simulink model "Droop_test2"  (R2024a)
settings: Solver=VariableStepAuto  StartTime=0.0  StopTime=1  RelTol=1e-3
InitFcn:
  |  if any(exist('rtifpga_mdlclblib', 'file') ~= 0), rtifpga_mdlclblib('Init', bdroot); end,
  | Ts  = 10e-6;
  | 
  | Vpeak = 170;
  | Vnom = Vpeak*sqrt(3)/sqrt(2);
  | Fnom = 60;
  | w_rad  = 2*pi*Fnom;
  | 
  | Vdc2 = 300;
  | 
  | % LC filter for DG1
  | L11 = 5e-03;
  | Cf1 = 30e-06;
  | Rc1 = 0.5;           % Damping series-resistor
  | RL1 = 0.9;        % Inductor ESR
  | L22=1e-12;
  | % LC filter for DG2
  | L12 = 5e-03;
  | Cf2 = 10e-06;
  | Rc2 = 0.5;           % Damping series-resistor
  | RL2 = 0.9;        % Inductor ESR
  | 
  | Pnom = 1000;
libraries: spsThreePhaseSeriesRLCBranchLib x5, spsabctoAlphaBetaZeroLib x4, spsGroundLib x3, spsFirstOrderFilterLib x2, spsThreePhaseVIMeasurementLib x2, spsabctodq0Lib x2, spsDCVoltageSourceLib x1, spsPLL3phLib x1, spsThreePhaseBreakerLib x1, spsUniversalBridgeLib x1, sps_lib x1
settings Model: Creator=azare  LastModifiedBy=nicho
settings OptimizationCC: ReuseModelBlockBuffer=off
settings RTWCC: GenCodeOnly=on  GPUComputeCapability=3.5
settings GRTTargetCC: OptimizeReductions=on

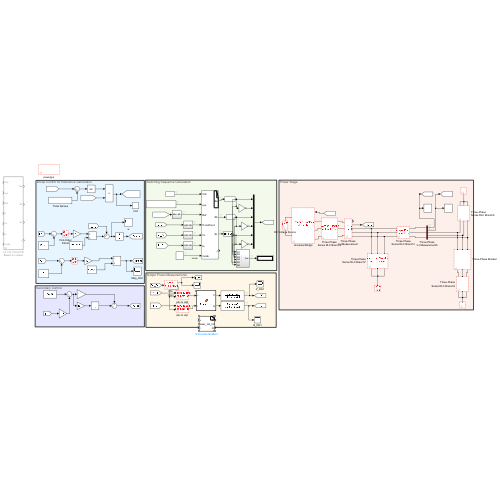
[thumbnail: Simulink's stored preview of the top-level diagram]
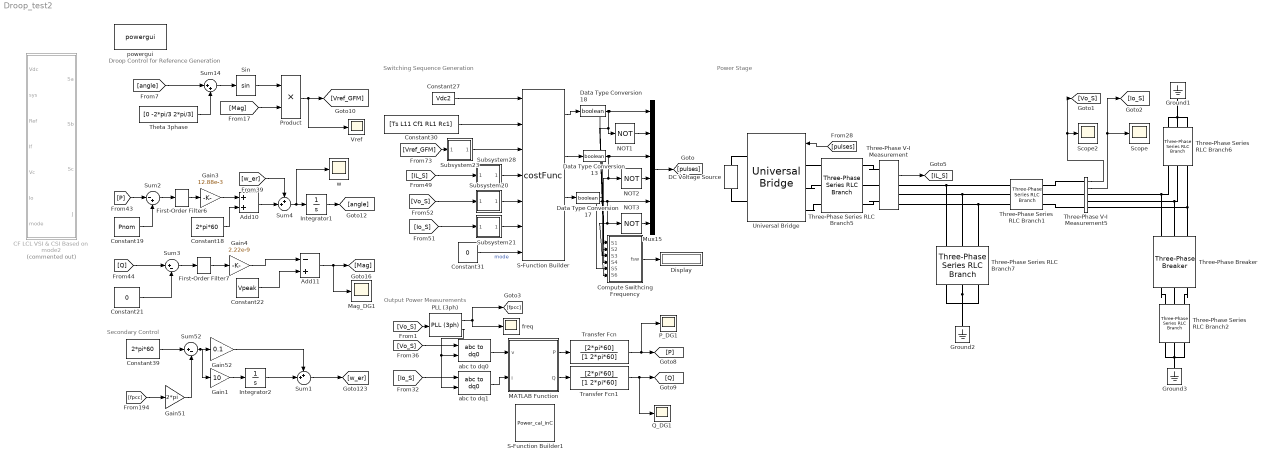
== system Droop_test2 ==
  note: Power Stage
  note: Output Power Measurements
  note: Switching Sequence Generation
  note: Droop Control for Reference Generation
  note: Secondary Control
  Add10 : Sum
  Add11 : Sum  Inputs=-+
  CF LCL VSI & CSI Based on mode2 : MATLAB Function  Commented=on  TreatAsAtomicUnit=on
  Compute Swithcing Frequency : Subsystem
  Constant18 : Constant  Value=2*pi*60
  Constant19 : Constant  Value=Pnom
  Constant21 : Constant  Value=0
  Constant22 : Constant  Value=Vpeak
  Constant27 : Constant  Value=Vdc2
  Constant30 : Constant  Value=[Ts L11 Cf1 RL1 Rc1]
  Constant31 : Constant  Value=0
  Constant39 : Constant  Value=2*pi*60
  DC Voltage Source : spsDCVoltageSourceLib/DC Voltage Source  Amplitude=Vdc2  Measurements=None
  Data Type Conversion13 : DataTypeConversion  OutDataTypeStr=boolean
  Data Type Conversion17 : DataTypeConversion  OutDataTypeStr=boolean
  Data Type Conversion18 : DataTypeConversion  OutDataTypeStr=boolean
  Display : Display
  First-Order Filter6 : spsFirstOrderFilterLib/First-Order Filter  FilterType=Lowpass  Tc=12.5e-3  Ts=0  Initialize=on  Vac_Init=[0, 0, 60]  Vdc_Init=0  PlotResponse=off  FreqRange="[0,  200,  1]"
  First-Order Filter7 : spsFirstOrderFilterLib/First-Order Filter  FilterType=Lowpass  Tc=12.5e-3  Ts=0  Initialize=on  Vac_Init=[0, 0, 60]  Vdc_Init=0  PlotResponse=off  FreqRange="[0,  200,  1]"
  Gain1 : Gain  Gain=10
  Gain3 : Gain  Gain=12.88e-3
  Gain4 : Gain  Gain=2.22e-9
  Gain51 : Gain  Gain=2*pi
  Gain52 : Gain  Gain=0.1
  Ground1 : spsGroundLib/Ground  LConnTagsString=a
  Ground2 : spsGroundLib/Ground  LConnTagsString=a
  Ground3 : spsGroundLib/Ground  LConnTagsString=a
  Integrator1 : Integrator
  Integrator2 : Integrator
  MATLAB Function : MATLAB Function  TreatAsAtomicUnit=on
  Mag_DG1 : Scope
  Mux15 : Mux  Inputs=6
  NOT1 : Logic  Operator=NOT  IconShape=distinctive  AllPortsSameDT=off  OutDataTypeStr=boolean
  NOT2 : Logic  Operator=NOT  IconShape=distinctive  AllPortsSameDT=off  OutDataTypeStr=boolean
  NOT3 : Logic  Operator=NOT  IconShape=distinctive  AllPortsSameDT=off  OutDataTypeStr=boolean
  PLL (3ph) : spsPLL3phLib/PLL (3ph)  Fmin=45  Par_Init=[0, 60]  ParK=[180, 3200, 1]  TcD=1e-4  MaxRateChangeFreq=12  FilterCutOffFreq=25  Ts=0  AGC=on
  P_DG1 : Scope
  Product : Product
  Q_DG1 : Scope
  S-Function Builder : S-Function  FunctionName=costFunc  SFunctionModules=costFunc_wrapper.c  SFunctionDeploymentMode=off  EnableBusSupport=off  mask(S-Function Builder){}
      mask help: Simulink:masks:SFunctionBuilder_MD
      mask init:
      | val = [[.9  0.75 0.75 1 1 .9 .9 1]',[1 1 0.75 0.75 .9 .9 1 .9]'];try , sys = get_param(gcb,'SfunBuilderFcnName');if isempty(sys), sys = get_param(gcb,'FunctionName'); end,catch, sys = get_param(gcb,'FunctionName'); end
      settings: CopyFcn=set_param(gcbh,'LinkStatus','none')  OpenFcn=sfunctionwizard(gcbh)
      mask Display:
      | plot(val(:,1),val(:,2))
      | disp(sys)
      | port_label('input',1,sprintf('%s', 'Vdc'),'interpreter','tex')
      | port_label('input',2,sprintf('%s', 'sys'),'interpreter','tex')
      | port_label('input',3,sprintf('%s', 'Ref'),'interpreter','tex')
      | port_label('input',4,sprintf('%s', 'If'),'interpreter','tex')
      | port_label('input',5,sprintf('%s', 'Vc'),'interpreter','tex')
      | port_label('input',6,sprintf('%s', 'Io'),'interpreter','tex')
      | port_label('input',7,sprintf('%s', 'mode'),'interpreter','tex')
      | port_label('output',1,sprintf('%s', 'Sa'),'interpreter','tex')
      | port_label('output',2,sprintf('%s', 'Sb'),'interpreter','tex')
      | port_label('output',3,sprintf('%s', 'Sc'),'interpreter','tex')
      | port_label('output',4,sprintf('%s', 'J'),'interpreter','tex')
  S-Function Builder1 : S-Function  FunctionName=Power_cal_inC  SFunctionModules=Power_cal_inC_wrapper.c  SFunctionDeploymentMode=off  EnableBusSupport=off  mask(S-Function Builder){}
      mask help: Simulink:masks:SFunctionBuilder_MD
      mask init: same as Droop_test2/S-Function Builder
      settings: CopyFcn=set_param(gcbh,'LinkStatus','none')  OpenFcn=sfunctionwizard(gcbh)
      mask Display: plot(val(:,1),val(:,2)),disp(sys),port_label('input',1,'v'),port_label('input',2,'i'),port_label('output',1,'P'),port_label('output',2,'Q')
  Scope : Scope
  Scope2 : Scope
  Sin : Trigonometry
  Subsystem20 : Subsystem
  Subsystem21 : Subsystem
  Subsystem23 : Subsystem
  Subsystem28 : Subsystem
  Sum1 : Sum  Inputs=++|
  Sum14 : Sum  Inputs=|++
  Sum2 : Sum  Inputs=|-+
  Sum3 : Sum  Inputs=|+-
  Sum4 : Sum  Inputs=++|
  Sum52 : Sum  Inputs=|+-
  Theta 3phase : Constant  Value=[0 -2*pi/3 2*pi/3]
  Three-Phase Series RLC Branch1 : spsThreePhaseSeriesRLCBranchLib/Three-Phase Series RLC Branch  LConnTagsString=A|B|C  RConnTagsString=A|B|C  BranchType=RL  Resistance=0.05  Inductance=0.5e-3  Capacitance=0  Measurements=None
  Three-Phase Series RLC Branch2 : spsThreePhaseSeriesRLCBranchLib/Three-Phase Series RLC Branch  LConnTagsString=A|B|C  RConnTagsString=A|B|C  BranchType=R  Resistance=43.35  Inductance=1e-3  Capacitance=10e-6  Measurements=None
  Three-Phase Series RLC Branch5 : spsThreePhaseSeriesRLCBranchLib/Three-Phase Series RLC Branch  LConnTagsString=A|B|C  RConnTagsString=A|B|C  BranchType=RL  Resistance=RL1  Inductance=L11  Capacitance=0  Measurements=None
  Three-Phase Series RLC Branch6 : spsThreePhaseSeriesRLCBranchLib/Three-Phase Series RLC Branch  LConnTagsString=A|B|C  RConnTagsString=A|B|C  BranchType=R  Resistance=43.35  Inductance=1e-3  Capacitance=10e-6  Measurements=None
  Three-Phase Series RLC Branch7 : spsThreePhaseSeriesRLCBranchLib/Three-Phase Series RLC Branch  LConnTagsString=A|B|C  RConnTagsString=A|B|C  BranchType=RC  Resistance=Rc1  Inductance=1e-3  Capacitance=Cf1  Measurements=None
  Three-Phase V-I Measurement : spsThreePhaseVIMeasurementLib/Three-Phase V-I Measurement  VoltageMeasurement=phase-to-ground  SetLabelV=off  LabelV=Vabc  Vpu=off  VpuLL=off  CurrentMeasurement=yes  SetLabelI=off  LabelI=Iabc  Ipu=off  Pbase=100e6  Vbase=500e3  OutputType=Complex  PhasorSimulation=off  PSBequivalent=0
  Three-Phase V-I Measurement5 : spsThreePhaseVIMeasurementLib/Three-Phase V-I Measurement  VoltageMeasurement=phase-to-ground  SetLabelV=off  LabelV=Vabc  Vpu=off  VpuLL=off  CurrentMeasurement=yes  SetLabelI=off  LabelI=Iabc  Ipu=off  Pbase=100e6  Vbase=500e3  OutputType=Complex  PhasorSimulation=off  PSBequivalent=0
  Three-Phase Breaker : spsThreePhaseBreakerLib/Three-Phase Breaker  InitialState=open  SwitchA=on  SwitchB=on  SwitchC=on  SwitchTimes=[4 8]  External=off  BreakerResistance=0.01  SnubberResistance=1e6  SnubberCapacitance=inf  Measurements=None
  Transfer Fcn : TransferFcn  Numerator=[2*pi*60]  Denominator=[1 2*pi*60]
  Transfer Fcn1 : TransferFcn  Numerator=[2*pi*60]  Denominator=[1 2*pi*60]
  Universal Bridge : spsUniversalBridgeLib/Universal Bridge  Arms=3  SnubberResistance=1e5  SnubberCapacitance=inf  Device=IGBT / Diodes  Ron=1e-3  Lon=0  ForwardVoltages="[  0  0  ]"  ForwardVoltage=0  GTOparameters=[ 10e-6 , 20e-6 ]  IGBTparameters=[ 1e-6 , 2e-6 ]  Measurements=None  Measurements_2=None  converterType=Rectifier
  Vref : Scope
  abc to dq0 : spsabctodq0Lib/abc to dq0  Alignment=90 degrees behind phase A axis
  abc to dq1 : spsabctodq0Lib/abc to dq0  Alignment=90 degrees behind phase A axis
  freq : Scope
  powergui : sps_lib/powergui  Priority=1  SimulationMode=Discrete  SampleTime=Ts  frequency=60  Iterations=50  frequencyindice=0  Pbase=100e6  ErrMax=1e-4  UnitsV=kV  UnitsW=MW  buscounter=0  FunctionMessages=off  echomessages=off  EnableUseOfTLC=off  CurrentSourceSwitches=off  DisableSnubberDevices=off  DisableRonSwitches=off  DisableVfSwitches=off  DisplayEquations=off  AutomaticDiscreteSolvers=off  SolverType=Tustin/Backward Euler (TBE)  Interpol=off  ExternalGateDelay=off  methode=off  Ts=100  x0status=blocks  SPID=on  SwTol=0  HookPort=off  NonlinearTolerance=1e-4  nMaxIteration=100  ContinueOnMaxIteration=off  RestoreLinks=warning  ResistiveCurrentMeasurement=off  Frange=[0:2:500]  Ylog=off  Xlog=on  ShowGrid=off  save=off  variable=ZData  structure=0  ZoomFFT=off  StartTime=0.0  cycles=1  DisplayStyle=1  fundamental=60  FreqAxis=off  MaxFrequency=1000  frequencyindicesteady=1  RmsSteady=1  display=off
  w : Scope
  wires:
  [Vo_S] -> Subsystem20/1(abc)
  S-Function Builder/2 -> Data Type Conversion13/1
  First-Order Filter6/1 -> Gain3/1
  Add11/1 -> Mag_DG1/1, [Mag]
  Gain4/1 -> Add11/1
  Constant18/1 -> Add10/2
  [IL_S] -> Subsystem28/1(abc)
  Gain3/1 -> Add10/1
  [Q] -> Sum3/1
  Subsystem23/1(ab) -> S-Function Builder/3
  Constant21/1 -> Sum3/2
  Constant19/1 -> Sum2/2
  S-Function Builder/3 -> Data Type Conversion17/1
  [Io_S] -> Subsystem21/1(abc)
  Integrator1/1 -> [angle]
  Constant27/1 -> S-Function Builder/1
  Constant31/1 -> S-Function Builder/7  "mode"
  Subsystem20/1(ab) -> S-Function Builder/5
  [P] -> Sum2/1
  Sum3/1 -> First-Order Filter7/1
  Subsystem28/1(ab) -> S-Function Builder/4
  Sum2/1 -> First-Order Filter6/1
  [Vref_GFM] -> Subsystem23/1(abc)
  Subsystem21/1(ab) -> S-Function Builder/6
  First-Order Filter7/1 -> Gain4/1
  Constant22/1 -> Add11/2
  Constant30/1 -> S-Function Builder/2
  Three-Phase V-I Measurement/2 -> [IL_S]
  [pulses] -> Universal Bridge/1
  Transfer Fcn1/1 -> Q_DG1/1, [Q]
  abc to dq1/1 -> MATLAB Function/2(i)
  Sum52/1 -> Gain1/1, Gain52/1
  [Io_S] -> abc to dq1/1
  Sin/1 -> Product/1
  Product/1 -> Vref/1, [Vref_GFM]
  Theta 3phase/1 -> Sum14/2
  Sum14/1 -> Sin/1
  Gain51/1 -> Sum52/2
  [fpcc] -> Gain51/1
  MATLAB Function/2(Q) -> Transfer Fcn1/1
  [Vo_S] -> abc to dq0/1
  MATLAB Function/1(P) -> Transfer Fcn/1
  abc to dq0/1 -> MATLAB Function/1(v)
  Transfer Fcn/1 -> P_DG1/1, [P]
  [angle] -> Sum14/1
  [Mag] -> Product/2
  Constant39/1 -> Sum52/1
  PLL (3ph)/2 -> abc to dq1/2, abc to dq0/2
  Three-Phase V-I Measurement5/1 -> [Vo_S], Scope2/1
  Three-Phase V-I Measurement5/2 -> [Io_S], Scope/1
  [w_er] -> Sum4/1
  Add10/1 -> Sum4/2
  Sum4/1 -> Integrator1/1, w/1
  [Vo_S] -> PLL (3ph)/1
  PLL (3ph)/1 -> freq/1, [fpcc]
  Sum1/1 -> [w_er]
  Gain1/1 -> Integrator2/1
  Integrator2/1 -> Sum1/2
  Gain52/1 -> Sum1/1
  Mux15/1 -> [pulses]
  Data Type Conversion17/1 -> Compute Swithcing Frequency/5(S5), Compute Swithcing Frequency/6(S6), NOT3/1, Mux15/5
  NOT3/1 -> Mux15/6
  Data Type Conversion18/1 -> Compute Swithcing Frequency/1(S1), Compute Swithcing Frequency/2(S2), NOT1/1, Mux15/1
  NOT1/1 -> Mux15/2
  Data Type Conversion13/1 -> Mux15/3, Compute Swithcing Frequency/3(S3), NOT2/1, Compute Swithcing Frequency/4(S4)
  NOT2/1 -> Mux15/4
  Compute Swithcing Frequency/1(fsw) -> Display/1
  S-Function Builder/1 -> Data Type Conversion18/1
  connections:
  Three-Phase V-I Measurement5/RConn3 -- Three-Phase Breaker/RConn3 -- Three-Phase Series RLC Branch6/LConn3
  Three-Phase Series RLC Branch7/RConn2 -- Ground2/LConn1 -- Three-Phase Series RLC Branch7/RConn3 -- Three-Phase Series RLC Branch7/RConn1
  Three-Phase V-I Measurement5/RConn2 -- Three-Phase Breaker/RConn2 -- Three-Phase Series RLC Branch6/LConn2
  Three-Phase V-I Measurement5/RConn1 -- Three-Phase Breaker/RConn1 -- Three-Phase Series RLC Branch6/LConn1
  Universal Bridge/LConn1 -- Three-Phase Series RLC Branch5/LConn1
  Three-Phase V-I Measurement/LConn3 -- Three-Phase Series RLC Branch5/RConn3
  Universal Bridge/LConn3 -- Three-Phase Series RLC Branch5/LConn3
  Three-Phase V-I Measurement/LConn1 -- Three-Phase Series RLC Branch5/RConn1
  Universal Bridge/LConn2 -- Three-Phase Series RLC Branch5/LConn2
  Three-Phase V-I Measurement/LConn2 -- Three-Phase Series RLC Branch5/RConn2
  DC Voltage Source/LConn1 -- Universal Bridge/RConn2
  DC Voltage Source/RConn1 -- Universal Bridge/RConn1
  Three-Phase Series RLC Branch6/RConn2 -- Three-Phase Series RLC Branch6/RConn3 -- Three-Phase Series RLC Branch6/RConn1 -- Ground1/LConn1
  Three-Phase V-I Measurement/RConn2 -- Three-Phase Series RLC Branch1/LConn2 -- Three-Phase Series RLC Branch7/LConn2
  Three-Phase V-I Measurement/RConn3 -- Three-Phase Series RLC Branch1/LConn3 -- Three-Phase Series RLC Branch7/LConn3
  Three-Phase V-I Measurement/RConn1 -- Three-Phase Series RLC Branch1/LConn1 -- Three-Phase Series RLC Branch7/LConn1
  Three-Phase Series RLC Branch1/RConn2 -- Three-Phase V-I Measurement5/LConn2
  Three-Phase Series RLC Branch1/RConn3 -- Three-Phase V-I Measurement5/LConn3
  Three-Phase Series RLC Branch1/RConn1 -- Three-Phase V-I Measurement5/LConn1
  Three-Phase Series RLC Branch2/RConn1 -- Three-Phase Series RLC Branch2/RConn3 -- Three-Phase Series RLC Branch2/RConn2 -- Ground3/LConn1
  Three-Phase Breaker/LConn1 -- Three-Phase Series RLC Branch2/LConn1
  Three-Phase Breaker/LConn2 -- Three-Phase Series RLC Branch2/LConn2
  Three-Phase Breaker/LConn3 -- Three-Phase Series RLC Branch2/LConn3

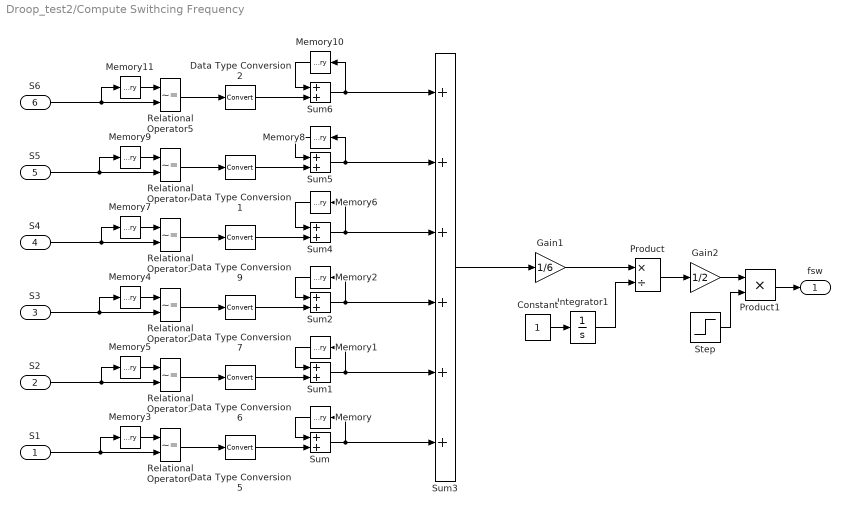
== system Droop_test2/Compute Swithcing Frequency ==
  S1 : Inport
  S2 : Inport  Port=2
  S3 : Inport  Port=3
  S4 : Inport  Port=4
  S5 : Inport  Port=5
  S6 : Inport  Port=6
  Constant : Constant
  Data Type Conversion{1..2,5..7,9} (6 alike) : DataTypeConversion  SaturateOnIntegerOverflow=off  RndMeth=Floor
  Gain1 : Gain  Gain=1/6  SaturateOnIntegerOverflow=on  OutDataTypeStr=Inherit: Same as input  ParamDataTypeStr=Inherit: Same as input
  Gain2 : Gain  Gain=1/2  SaturateOnIntegerOverflow=on  OutDataTypeStr=Inherit: Same as input  ParamDataTypeStr=Inherit: Same as input
  Integrator1 : Integrator  InitialCondition=0.000000000000000000001
  Memory{,1..11} (12 alike) : Memory
  Product : Product  Inputs=*/  SaturateOnIntegerOverflow=on
  Product1 : Product
  Relational Operator{1..6} (6 alike) : RelationalOperator  Operator=~=
  Step : Step  Time=Ts  SampleTime=0
  Sum{,1..2,4..6} (6 alike) : Sum  InputSameDT=on  SaturateOnIntegerOverflow=on  OutDataTypeStr=Inherit: Same as first input
  Sum3 : Sum  Inputs=++++++  SaturateOnIntegerOverflow=on
  fsw : Outport  VectorParamsAs1DForOutWhenUnconnected=off
  wires:
  Memory3/1 -> Relational Operator6/1
  Relational Operator6/1 -> Data Type Conversion5/1
  S1/1 -> Relational Operator6/2, Memory3/1
  Memory5/1 -> Relational Operator1/1
  Relational Operator1/1 -> Data Type Conversion6/1
  Sum1/1 -> Sum3/5, Memory1/1
  Memory1/1 -> Sum1/1
  S2/1 -> Relational Operator1/2, Memory5/1
  Memory4/1 -> Relational Operator2/1
  Relational Operator2/1 -> Data Type Conversion7/1
  Sum2/1 -> Sum3/4, Memory2/1
  Memory2/1 -> Sum2/1
  S3/1 -> Relational Operator2/2, Memory4/1
  Sum3/1 -> Gain1/1
  Gain1/1 -> Product/1
  Integrator1/1 -> Product/2
  Constant/1 -> Integrator1/1
  Product/1 -> Gain2/1
  Memory7/1 -> Relational Operator3/1
  Relational Operator3/1 -> Data Type Conversion9/1
  Sum4/1 -> Sum3/3, Memory6/1
  Memory6/1 -> Sum4/1
  S4/1 -> Relational Operator3/2, Memory7/1
  Data Type Conversion7/1 -> Sum2/2
  Data Type Conversion9/1 -> Sum4/2
  Data Type Conversion6/1 -> Sum1/2
  Memory/1 -> Sum/1
  Data Type Conversion5/1 -> Sum/2
  Data Type Conversion2/1 -> Sum6/2
  Data Type Conversion1/1 -> Sum5/2
  S6/1 -> Memory11/1, Relational Operator5/2
  Memory10/1 -> Sum6/1
  Sum6/1 -> Sum3/1, Memory10/1
  Relational Operator5/1 -> Data Type Conversion2/1
  Memory11/1 -> Relational Operator5/1
  S5/1 -> Memory9/1, Relational Operator4/2
  Memory8/1 -> Sum5/1
  Sum5/1 -> Sum3/2, Memory8/1
  Relational Operator4/1 -> Data Type Conversion1/1
  Memory9/1 -> Relational Operator4/1
  Sum/1 -> Sum3/6, Memory/1
  Product1/1 -> fsw/1
  Step/1 -> Product1/2
  Gain2/1 -> Product1/1

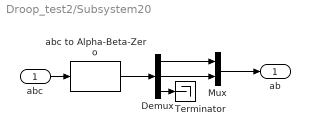
== system Droop_test2/Subsystem20 ==
  abc : Inport
  Demux : Demux  Outputs=3
  Mux : Mux  Inputs=2
  Terminator : Terminator
  abc to Alpha-Beta-Zero : spsabctoAlphaBetaZeroLib/abc to Alpha-Beta-Zero
  ab : Outport
  wires:
  Demux/2 -> Mux/2
  abc to Alpha-Beta-Zero/1 -> Demux/1
  Mux/1 -> ab/1
  Demux/1 -> Mux/1
  abc/1 -> abc to Alpha-Beta-Zero/1
  Demux/3 -> Terminator/1

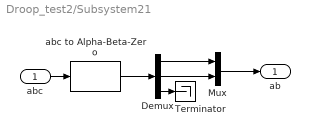
== system Droop_test2/Subsystem21 ==
  abc : Inport
  Demux : Demux  Outputs=3
  Mux : Mux  Inputs=2
  Terminator : Terminator
  abc to Alpha-Beta-Zero : spsabctoAlphaBetaZeroLib/abc to Alpha-Beta-Zero
  ab : Outport
  wires:
  Demux/3 -> Terminator/1
  abc/1 -> abc to Alpha-Beta-Zero/1
  Demux/1 -> Mux/1
  Mux/1 -> ab/1
  abc to Alpha-Beta-Zero/1 -> Demux/1
  Demux/2 -> Mux/2

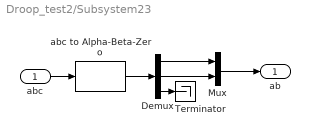
== system Droop_test2/Subsystem23 ==
  abc : Inport
  Demux : Demux  Outputs=3
  Mux : Mux  Inputs=2
  Terminator : Terminator
  abc to Alpha-Beta-Zero : spsabctoAlphaBetaZeroLib/abc to Alpha-Beta-Zero
  ab : Outport
  wires:
  Demux/2 -> Mux/2
  abc to Alpha-Beta-Zero/1 -> Demux/1
  Mux/1 -> ab/1
  Demux/1 -> Mux/1
  abc/1 -> abc to Alpha-Beta-Zero/1
  Demux/3 -> Terminator/1

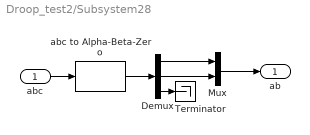
== system Droop_test2/Subsystem28 ==
  abc : Inport
  Demux : Demux  Outputs=3
  Mux : Mux  Inputs=2
  Terminator : Terminator
  abc to Alpha-Beta-Zero : spsabctoAlphaBetaZeroLib/abc to Alpha-Beta-Zero
  ab : Outport
  wires:
  Demux/3 -> Terminator/1
  abc/1 -> abc to Alpha-Beta-Zero/1
  Demux/1 -> Mux/1
  Mux/1 -> ab/1
  abc to Alpha-Beta-Zero/1 -> Demux/1
  Demux/2 -> Mux/2

== matlab function Droop_test2/MATLAB Function ==
  data: v input; P output; i input; Q output
function [P,Q] = Power_cal(v,i)

P=3*(0.5 * (v(1)*i(1) + v(2)*i(2)) );
Q=3*(0.5 * (v(1)*i(2) - v(2)*i(1)) );

== matlab function Droop_test2/CF LCL VSI & CSI Based on mode2 ==
  settings: updateMethod=DISCRETE
  data: Vdc input; sys input; Ref input; If input; Vc input; Io input; Sa output; Sb output; Sc output; mode input; J output
 function [Sa, Sb, Sc, J] = fcn(Vdc, sys, Ref, If, Vc, Io, mode)

Sa = 0;
Sb = 0;
Sc = 0;

xout  = 0;
J     = 0;
J_out = 1e9;

Ts  = sys(1); 
Lf  = sys(2);
Cf  = sys(3); 
Rf  = sys(4);      % Inductor ESR 
Rc  = sys(5);

refa = Ref(1);          refb = Ref(2);
Vca   = Vc(1);         Vcb = Vc(2);
Ioa   = Io(1);           Iob = Io(2);
ILa   = If(1);            ILb = If(2);

VSI = 0; CSI = 0;  % Initialize Modes for Cost Function
Mode = VSI;        % Select Operation Mode

if mode == 0 
    VSI = 1; CSI = 0; 
elseif mode > 0
    VSI = 0; CSI = 1;
end
% disp(CSI); disp(VSI);

% A = [-R/L -1/L;1/Cf 0   ;  ...
%      Rc/Cf       0        -Rc/Cf;  ...
%      0        1/Lt    -Rt/Lt ];
% 
% B = [1/Lf; 0; 0];
% 
% D = [0 0;0 -1/Lf];
A = [-Rf/Lf -1/Lf;1/Cf 0];
B = [1/Lf 0;0 -1/Cf];

I  = eye(2);
Ad = expm(A.*Ts);
Bd = A\(Ad - I);
% Dd = inv(A)*(Ad - I)*D;

% Voltage vectors
v0 =  0;
v1 =  2/3 *Vdc;
v2 =  1/3*Vdc + 1j*sqrt(3)/3*Vdc;
v3 = -1/3*Vdc + 1j*sqrt(3)/3*Vdc;
v4 = -2/3*Vdc;
v5 = -1/3*Vdc - 1j*sqrt(3)/3*Vdc;
v6 =  1/3*Vdc - 1j*sqrt(3)/3*Vdc;
v7 =  0;
Vinv = [v0 v1 v2 v3 v4 v5 v6 v7];

states = [0 0 0; 1 0 0; 1 1 0; 0 1 0; ...
          0 1 1; 0 0 1; 1 0 1; 1 1 1];

% Avoid Error xout = 0 out of range [1,8]
% if xout == 0, xout = 1; end

for i = 1:8
    
% i-th voltage vector for current prediction
 Vinva = real(Vinv(i));  
 Vinvb = imag(Vinv(i));

% For alpha 
% x= Ad*[ILa;Vca;Ioa] + Bd*[Vinva]; + Dd*[Voa];
x= Ad*[ILa;Vca] + Bd*[Vinva;Ioa]; 
V_k1a = x(2);

% For Beta 
% y= Ad*[ILb;Vcb;Iob] + Bd*[Vinvb] + Dd*[Vob];
y= Ad*[ILb;Vcb] + Bd*[Vinvb;Iob];
V_k1b = y(2);

   

J = VSI*((refa - V_k1a)^2 + (refb - V_k1b)^2);

if ( J < J_out)
      J_out = J;
       xout = i;
end
  
end

 Sa = states(xout,1);
 Sb = states(xout,2);
 Sc = states(xout,3);
